simulink model "float_point"  (R2022a)
settings: Solver=VariableStepAuto  StartTime=0.0  StopTime=10.0  RelTol=1e-3
settings Model: Creator=User  LastModifiedBy=User

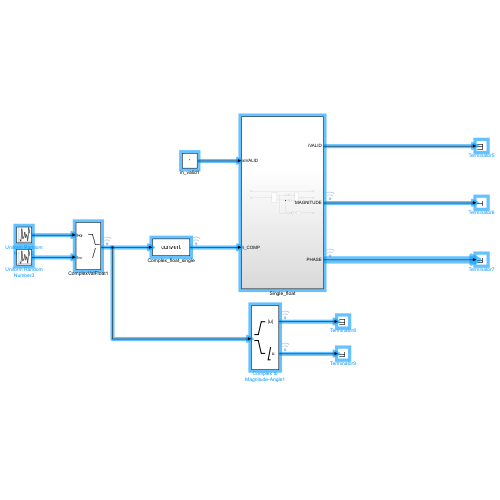
[thumbnail: Simulink's stored preview of the top-level diagram]
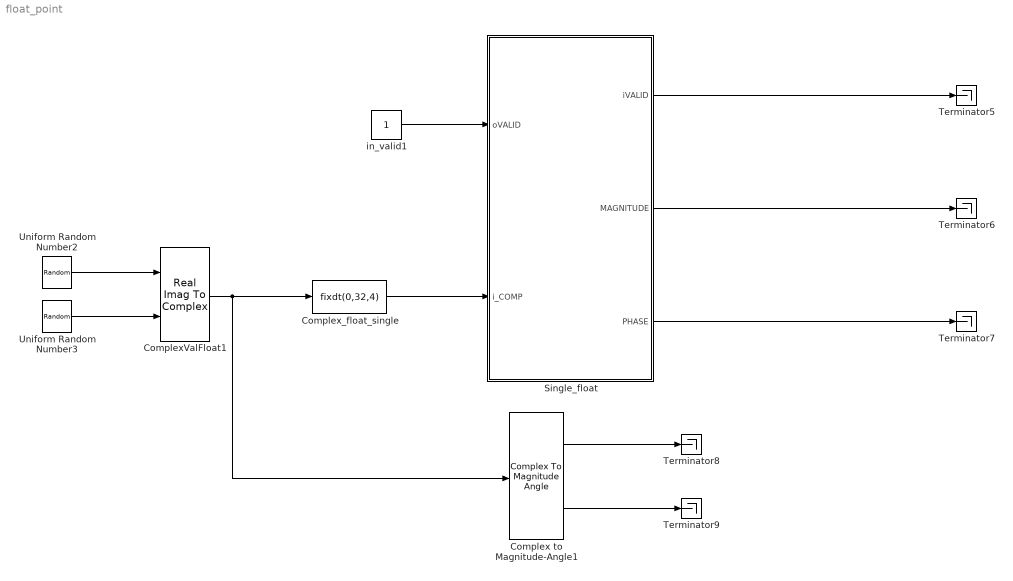
== system float_point ==
  Complex to Magnitude-Angle1 : ComplexToMagnitudeAngle
  ComplexValFloat1 : RealImagToComplex
  Complex_float_single : DataTypeConversion  OutDataTypeStr=fixdt(0,32,4)  RndMeth=Round  SaturateOnIntegerOverflow=off
  Single_float : Subsystem
  Terminator{5..9} (5 alike) : Terminator
  Uniform Random Number2 : UniformRandomNumber  Minimum=0  Maximum=2 ^(28) - 1  Seed=28  SampleTime=1
  Uniform Random Number3 : UniformRandomNumber  Minimum=0  Maximum=2 ^(28) - 1  Seed=28  SampleTime=1
  in_valid1 : Constant  OutDataTypeStr=boolean  SampleTime=1
  wires:
  Single_float/1(iVALID) -> Terminator5/1
  Complex to Magnitude-Angle1/2 -> Terminator9/1
  Complex to Magnitude-Angle1/1 -> Terminator8/1
  ComplexValFloat1/1 -> Complex to Magnitude-Angle1/1, Complex_float_single/1
  in_valid1/1 -> Single_float/1(oVALID)
  Uniform Random Number2/1 -> ComplexValFloat1/1
  Single_float/2(MAGNITUDE) -> Terminator6/1
  Uniform Random Number3/1 -> ComplexValFloat1/2
  Complex_float_single/1 -> Single_float/2(i_COMP)
  Single_float/3(PHASE) -> Terminator7/1

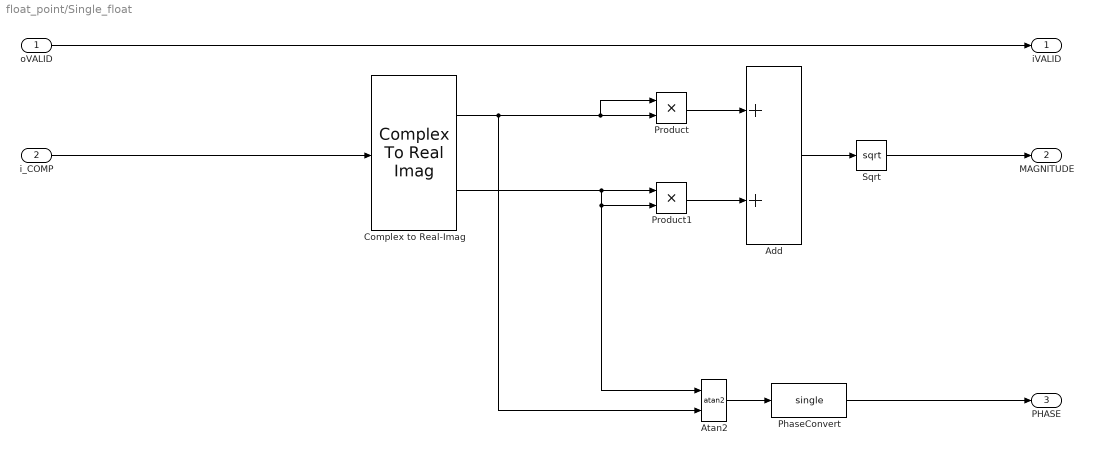
== system float_point/Single_float ==
  oVALID : Inport  OutDataTypeStr=boolean
  i_COMP : Inport  Port=2
  Add : Sum
  Atan2 : Trigonometry  Operator=atan2  ApproximationMethod=CORDIC
  Complex to Real-Imag : ComplexToRealImag
  PhaseConvert : DataTypeConversion  OutDataTypeStr=single  RndMeth=Round  SaturateOnIntegerOverflow=off
  Product : Product
  Product1 : Product
  Sqrt : Sqrt  OutDataTypeStr=single
  iVALID : Outport
  MAGNITUDE : Outport  Port=2
  PHASE : Outport  Port=3
  wires:
  Add/1 -> Sqrt/1
  Product/1 -> Add/1
  Sqrt/1 -> MAGNITUDE/1
  Product1/1 -> Add/2
  Atan2/1 -> PhaseConvert/1
  i_COMP/1 -> Complex to Real-Imag/1
  oVALID/1 -> iVALID/1
  PhaseConvert/1 -> PHASE/1
  Complex to Real-Imag/2 -> Atan2/1, Product1/2, Product1/1
  Complex to Real-Imag/1 -> Product/1, Product/2, Atan2/2
